simulink model "espresso_pid_wired_model_2023a"  (R2023a)
settings: Solver=VariableStepAuto  StartTime=0.0  StopTime=10  RelTol=1e-3
libraries: simulink x4, slpidlib x3
settings Model: Creator=nikonatsoulas  LastModifiedBy=Lillian K

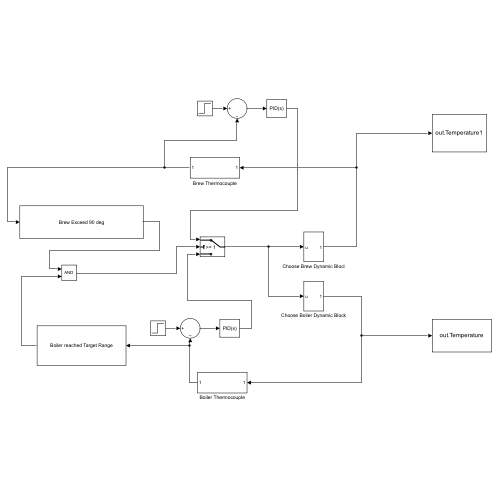
[thumbnail: Simulink's stored preview of the top-level diagram]
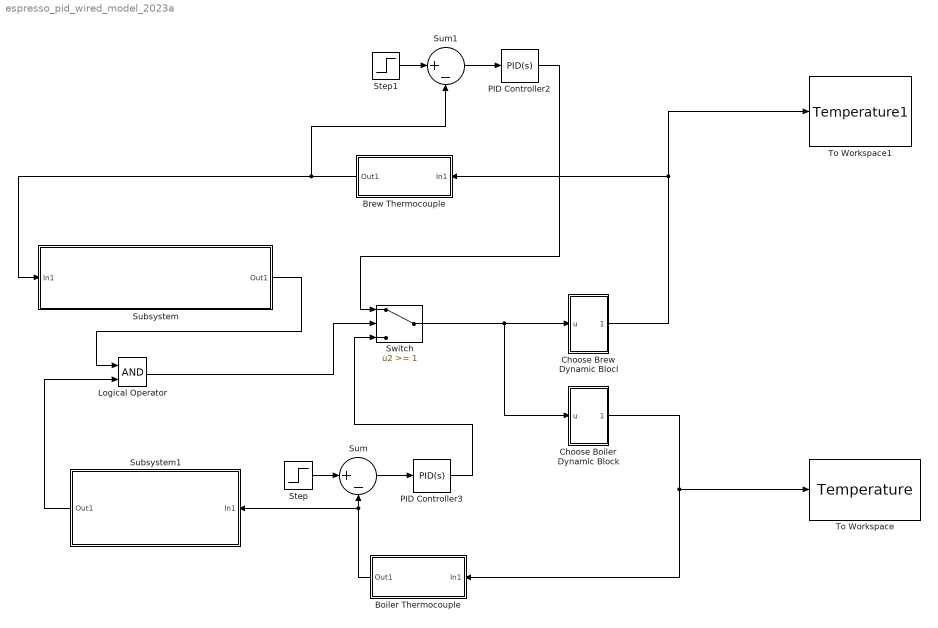
== system espresso_pid_wired_model_2023a ==
  Boiler Thermocouple : Subsystem
  Brew Thermocouple : Subsystem
  Choose Boiler Dynamic Block : Subsystem
  Choose Brew Dynamic Blocl : Subsystem
  Logical Operator : Logic  AllPortsSameDT=off  OutDataTypeStr=boolean
  PID Controller2 : slpidlib/PID Controller  Controller=PID  Form=Parallel  TimeDomain=Continuous-time  UseExternalTs=off  SampleTime=-1  IntegratorMethod=Forward Euler  FilterMethod=Forward Euler  ControllerParametersSource=internal  P=1.2  I=0.078  UseKiTs=off  D=0.08  N=100  UseFilter=on  TunerSelectOption=Transfer Function Based (PID Tuner App)  InitialConditionSource=internal  InitialConditionForIntegrator=0  InitialConditionForFilter=0  DifferentiatorICPrevScaledInput=0  ExternalReset=none  TrackingMode=off  Kt=1  LimitOutput=off  SatLimitsSource=internal  UpperSaturationLimit=inf  LowerSaturationLimit=-inf  LinearizeAsGain=on  AntiWindupMode=none  Kb=1  LimitIntegrator=off  UpperIntegratorSaturationLimit=inf  LowerIntegratorSaturationLimit=-inf  POutMin=[]  POutMax=[]  IOutMin=[]  IOutMax=[]  DOutMin=[]  DOutMax=[]  NOutMin=[]  NOutMax=[]  SumOutMin=[]  SumOutMax=[]  SaturationOutMin=[]  SaturationOutMax=[]  PParamMin=[]  PParamMax=[]  IParamMin=[]  IParamMax=[]  DParamMin=[]  DParamMax=[]  NParamMin=[]  NParamMax=[]  KbParamMin=[]  KbParamMax=[]  KtParamMin=[]  KtParamMax=[]  KbOutMin=[]  KbOutMax=[]  KtOutMin=[]  KtOutMax=[]  IntegratorOutMin=[]  IntegratorOutMax=[]  FilterOutMin=[]  FilterOutMax=[]  SumI1OutMin=[]  SumI1OutMax=[]  SumI2OutMin=[]  SumI2OutMax=[]  SumI3OutMin=[]  SumI3OutMax=[]  SumI4OutMin=[]  SumI4OutMax=[]  SumDOutMin=[]  SumDOutMax=[]  DifferentiatorOutMin=[]  DifferentiatorOutMax=[]  FilterDiffOutCoefMin=[]  FilterDiffOutCoefMax=[]  ReciprocalOutMin=[]  ReciprocalOutMax=[]  SumDenOutMin=[]  SumDenOutMax=[]  SumNumOutMin=[]  SumNumOutMax=[]  DivideOutMin=[]  DivideOutMax=[]  UdiffTsProdOutMin=[]  UdiffTsProdOutMax=[]  NTsProdOutMin=[]  NTsProdOutMax=[]  UintegralTsProdOutMin=[]  UintegralTsProdOutMax=[]  UngainTsProdOutMin=[]  UngainTsProdOutMax=[]  ClampingZeroOutDataTypeStr=Inherit: Inherit via back propagation  ClampingZeroOutMin=[]  ClampingZeroOutMax=[]  FilterDenConstantOutDataTypeStr=Inherit: Inherit via back propagation  FilterDenConstantOutMin=[]  FilterDenConstantOutMax=[]  PCopyOutDataTypeStr=Inherit: Inherit via back propagation  PCopyOutMin=[]  PCopyOutMax=[]  NCopyOutDataTypeStr=Inherit: Inherit via back propagation  NCopyOutMin=[]  NCopyOutMax=[]  IntegratorContinuousStateAttributes=''  IntegratorStateMustResolveToSignalObject=off  IntegratorRTWStateStorageClass=Auto  FilterContinuousStateAttributes=''  FilterStateMustResolveToSignalObject=off  FilterRTWStateStorageClass=Auto  ParallelPVariant=InternalParameters  IdealPVariant=Disabled  IVariant=InternalParameters  DVariant=InternalParameters  IntegratorVariant=Continuous  SatVariant=Disabled  AWVariant=Passthrough  PCopyVariant=Disabled  TRVariant=Disabled  FdbkBlocksVariant=Forward  IdealPFdbkVariant=Disabled  SatFdbkVariant=Disabled  DerivativeFilterVariant=ContFilter  NVariant=InternalParameters  NCopyVariant=Disabled  FilterICVariant=InternalICsFilter  IntegratorICVariant=InternalICs  ExternalResetVariant=Disabled  TRSumVariant=Passthrough  SumFdbkVariant=Disabled  SumVariant=Sum_PID  TsampFilterVariant=InternalTs  TsampNgainVariant=Passthrough  TsampIntegralVariant=Disabled_SignalSpec  ExternalSaturationOutDataTypeStr=Inherit: Same as second input
  PID Controller3 : slpidlib/PID Controller  Controller=PID  Form=Parallel  TimeDomain=Continuous-time  UseExternalTs=off  SampleTime=-1  IntegratorMethod=Forward Euler  FilterMethod=Forward Euler  ControllerParametersSource=internal  P=1.2  I=0.078  UseKiTs=off  D=0.08  N=100  UseFilter=on  TunerSelectOption=Transfer Function Based (PID Tuner App)  InitialConditionSource=internal  InitialConditionForIntegrator=0  InitialConditionForFilter=0  DifferentiatorICPrevScaledInput=0  ExternalReset=none  TrackingMode=off  Kt=1  LimitOutput=off  SatLimitsSource=internal  UpperSaturationLimit=inf  LowerSaturationLimit=-inf  LinearizeAsGain=on  AntiWindupMode=none  Kb=1  LimitIntegrator=off  UpperIntegratorSaturationLimit=inf  LowerIntegratorSaturationLimit=-inf  POutMin=[]  POutMax=[]  IOutMin=[]  IOutMax=[]  DOutMin=[]  DOutMax=[]  NOutMin=[]  NOutMax=[]  SumOutMin=[]  SumOutMax=[]  SaturationOutMin=[]  SaturationOutMax=[]  PParamMin=[]  PParamMax=[]  IParamMin=[]  IParamMax=[]  DParamMin=[]  DParamMax=[]  NParamMin=[]  NParamMax=[]  KbParamMin=[]  KbParamMax=[]  KtParamMin=[]  KtParamMax=[]  KbOutMin=[]  KbOutMax=[]  KtOutMin=[]  KtOutMax=[]  IntegratorOutMin=[]  IntegratorOutMax=[]  FilterOutMin=[]  FilterOutMax=[]  SumI1OutMin=[]  SumI1OutMax=[]  SumI2OutMin=[]  SumI2OutMax=[]  SumI3OutMin=[]  SumI3OutMax=[]  SumI4OutMin=[]  SumI4OutMax=[]  SumDOutMin=[]  SumDOutMax=[]  DifferentiatorOutMin=[]  DifferentiatorOutMax=[]  FilterDiffOutCoefMin=[]  FilterDiffOutCoefMax=[]  ReciprocalOutMin=[]  ReciprocalOutMax=[]  SumDenOutMin=[]  SumDenOutMax=[]  SumNumOutMin=[]  SumNumOutMax=[]  DivideOutMin=[]  DivideOutMax=[]  UdiffTsProdOutMin=[]  UdiffTsProdOutMax=[]  NTsProdOutMin=[]  NTsProdOutMax=[]  UintegralTsProdOutMin=[]  UintegralTsProdOutMax=[]  UngainTsProdOutMin=[]  UngainTsProdOutMax=[]  ClampingZeroOutDataTypeStr=Inherit: Inherit via back propagation  ClampingZeroOutMin=[]  ClampingZeroOutMax=[]  FilterDenConstantOutDataTypeStr=Inherit: Inherit via back propagation  FilterDenConstantOutMin=[]  FilterDenConstantOutMax=[]  PCopyOutDataTypeStr=Inherit: Inherit via back propagation  PCopyOutMin=[]  PCopyOutMax=[]  NCopyOutDataTypeStr=Inherit: Inherit via back propagation  NCopyOutMin=[]  NCopyOutMax=[]  IntegratorContinuousStateAttributes=''  IntegratorStateMustResolveToSignalObject=off  IntegratorRTWStateStorageClass=Auto  FilterContinuousStateAttributes=''  FilterStateMustResolveToSignalObject=off  FilterRTWStateStorageClass=Auto  ParallelPVariant=InternalParameters  IdealPVariant=Disabled  IVariant=InternalParameters  DVariant=InternalParameters  IntegratorVariant=Continuous  SatVariant=Disabled  AWVariant=Passthrough  PCopyVariant=Disabled  TRVariant=Disabled  FdbkBlocksVariant=Forward  IdealPFdbkVariant=Disabled  SatFdbkVariant=Disabled  DerivativeFilterVariant=ContFilter  NVariant=InternalParameters  NCopyVariant=Disabled  FilterICVariant=InternalICsFilter  IntegratorICVariant=InternalICs  ExternalResetVariant=Disabled  TRSumVariant=Passthrough  SumFdbkVariant=Disabled  SumVariant=Sum_PID  TsampFilterVariant=InternalTs  TsampNgainVariant=Passthrough  TsampIntegralVariant=Disabled_SignalSpec  ExternalSaturationOutDataTypeStr=Inherit: Same as second input
  Step : Step  After=65  SampleTime=0
  Step1 : Step  SampleTime=0
  Subsystem : Subsystem
      mask Display: disp('Brew Exceed 90 deg')
  Subsystem1 : Subsystem
      mask Display: disp('Boiler reached Target Range')
  Sum : Sum  Inputs=|+-
  Sum1 : Sum  Inputs=|+-
  Switch : Switch  Threshold=1  SaturateOnIntegerOverflow=off  InputSameDT=off
  To Workspace : ToWorkspace  VariableName=Temperature  SaveFormat=Timeseries  SampleTime=-1
  To Workspace1 : ToWorkspace  VariableName=Temperature1  SaveFormat=Timeseries  SampleTime=-1
  wires:
  Step/1 -> Sum/1
  Boiler Thermocouple/1(Out1) -> Sum/2, Subsystem1/1(In1)
  Step1/1 -> Sum1/1
  Brew Thermocouple/1(Out1) -> Sum1/2, Subsystem/1(In1)
  PID Controller2/1 -> Switch/1
  PID Controller3/1 -> Switch/3
  Logical Operator/1 -> Switch/2
  Sum/1 -> PID Controller3/1
  Switch/1 -> Choose Brew Dynamic Blocl/1(u), Choose Boiler Dynamic Block/1(u)
  Sum1/1 -> PID Controller2/1
  Choose Boiler Dynamic Block/1(Out1) -> Boiler Thermocouple/1(In1), To Workspace/1
  Choose Brew Dynamic Blocl/1(Out1) -> To Workspace1/1, Brew Thermocouple/1(In1)
  Subsystem/1(Out1) -> Logical Operator/1
  Subsystem1/1(Out1) -> Logical Operator/2

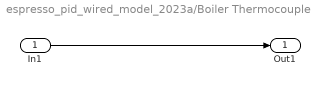
== system espresso_pid_wired_model_2023a/Boiler Thermocouple ==
  In1 : Inport
  Out1 : Outport
  wires:
  In1/1 -> Out1/1

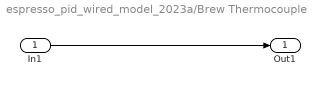
== system espresso_pid_wired_model_2023a/Brew Thermocouple ==
  In1 : Inport
  Out1 : Outport
  wires:
  In1/1 -> Out1/1

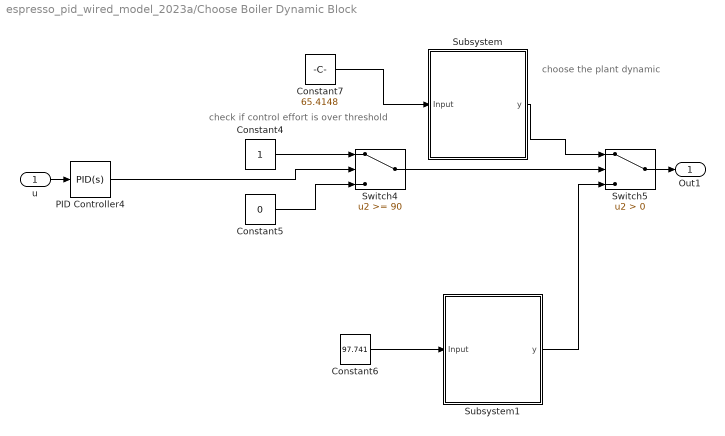
== system espresso_pid_wired_model_2023a/Choose Boiler Dynamic Block ==
  note: choose the plant dynamic
  note: check if control effort is over threshold
  u : Inport
  Constant4 : Constant
  Constant5 : Constant  Value=0
  Constant6 : Constant  Value=97.741
  Constant7 : Constant  Value=65.4148
  PID Controller4 : slpidlib/PID Controller  Controller=PID  Form=Parallel  TimeDomain=Continuous-time  UseExternalTs=off  SampleTime=-1  IntegratorMethod=Forward Euler  FilterMethod=Forward Euler  ControllerParametersSource=internal  P=1.2  I=0.078  UseKiTs=off  D=0.08  N=100  UseFilter=on  TunerSelectOption=Transfer Function Based (PID Tuner App)  InitialConditionSource=internal  InitialConditionForIntegrator=0  InitialConditionForFilter=0  DifferentiatorICPrevScaledInput=0  ExternalReset=none  TrackingMode=off  Kt=1  LimitOutput=off  SatLimitsSource=internal  UpperSaturationLimit=inf  LowerSaturationLimit=-inf  LinearizeAsGain=on  AntiWindupMode=none  Kb=1  LimitIntegrator=off  UpperIntegratorSaturationLimit=inf  LowerIntegratorSaturationLimit=-inf  POutMin=[]  POutMax=[]  IOutMin=[]  IOutMax=[]  DOutMin=[]  DOutMax=[]  NOutMin=[]  NOutMax=[]  SumOutMin=[]  SumOutMax=[]  SaturationOutMin=[]  SaturationOutMax=[]  PParamMin=[]  PParamMax=[]  IParamMin=[]  IParamMax=[]  DParamMin=[]  DParamMax=[]  NParamMin=[]  NParamMax=[]  KbParamMin=[]  KbParamMax=[]  KtParamMin=[]  KtParamMax=[]  KbOutMin=[]  KbOutMax=[]  KtOutMin=[]  KtOutMax=[]  IntegratorOutMin=[]  IntegratorOutMax=[]  FilterOutMin=[]  FilterOutMax=[]  SumI1OutMin=[]  SumI1OutMax=[]  SumI2OutMin=[]  SumI2OutMax=[]  SumI3OutMin=[]  SumI3OutMax=[]  SumI4OutMin=[]  SumI4OutMax=[]  SumDOutMin=[]  SumDOutMax=[]  DifferentiatorOutMin=[]  DifferentiatorOutMax=[]  FilterDiffOutCoefMin=[]  FilterDiffOutCoefMax=[]  ReciprocalOutMin=[]  ReciprocalOutMax=[]  SumDenOutMin=[]  SumDenOutMax=[]  SumNumOutMin=[]  SumNumOutMax=[]  DivideOutMin=[]  DivideOutMax=[]  UdiffTsProdOutMin=[]  UdiffTsProdOutMax=[]  NTsProdOutMin=[]  NTsProdOutMax=[]  UintegralTsProdOutMin=[]  UintegralTsProdOutMax=[]  UngainTsProdOutMin=[]  UngainTsProdOutMax=[]  ClampingZeroOutDataTypeStr=Inherit: Inherit via back propagation  ClampingZeroOutMin=[]  ClampingZeroOutMax=[]  FilterDenConstantOutDataTypeStr=Inherit: Inherit via back propagation  FilterDenConstantOutMin=[]  FilterDenConstantOutMax=[]  PCopyOutDataTypeStr=Inherit: Inherit via back propagation  PCopyOutMin=[]  PCopyOutMax=[]  NCopyOutDataTypeStr=Inherit: Inherit via back propagation  NCopyOutMin=[]  NCopyOutMax=[]  IntegratorContinuousStateAttributes=''  IntegratorStateMustResolveToSignalObject=off  IntegratorRTWStateStorageClass=Auto  FilterContinuousStateAttributes=''  FilterStateMustResolveToSignalObject=off  FilterRTWStateStorageClass=Auto  ParallelPVariant=InternalParameters  IdealPVariant=Disabled  IVariant=InternalParameters  DVariant=InternalParameters  IntegratorVariant=Continuous  SatVariant=Disabled  AWVariant=Passthrough  PCopyVariant=Disabled  TRVariant=Disabled  FdbkBlocksVariant=Forward  IdealPFdbkVariant=Disabled  SatFdbkVariant=Disabled  DerivativeFilterVariant=ContFilter  NVariant=InternalParameters  NCopyVariant=Disabled  FilterICVariant=InternalICsFilter  IntegratorICVariant=InternalICs  ExternalResetVariant=Disabled  TRSumVariant=Passthrough  SumFdbkVariant=Disabled  SumVariant=Sum_PID  TsampFilterVariant=InternalTs  TsampNgainVariant=Passthrough  TsampIntegralVariant=Disabled_SignalSpec  ExternalSaturationOutDataTypeStr=Inherit: Same as second input
  Subsystem : Subsystem
      mask Display: disp('Full 40 A to Brew')
  Subsystem1 : Subsystem
      mask Display: disp('0 A to Brew')
  Switch4 : Switch  Threshold=90  SaturateOnIntegerOverflow=off  InputSameDT=off
  Switch5 : Switch  Criteria=u2 > Threshold  SaturateOnIntegerOverflow=off  InputSameDT=off
  Out1 : Outport
  wires:
  Constant5/1 -> Switch4/3
  Switch4/1 -> Switch5/2
  PID Controller4/1 -> Switch4/2
  Constant6/1 -> Subsystem1/1(Input)
  Constant7/1 -> Subsystem/1(Input)
  Constant4/1 -> Switch4/1
  Subsystem/1(y) -> Switch5/1
  Subsystem1/1(y) -> Switch5/3
  Switch5/1 -> Out1/1
  u/1 -> PID Controller4/1

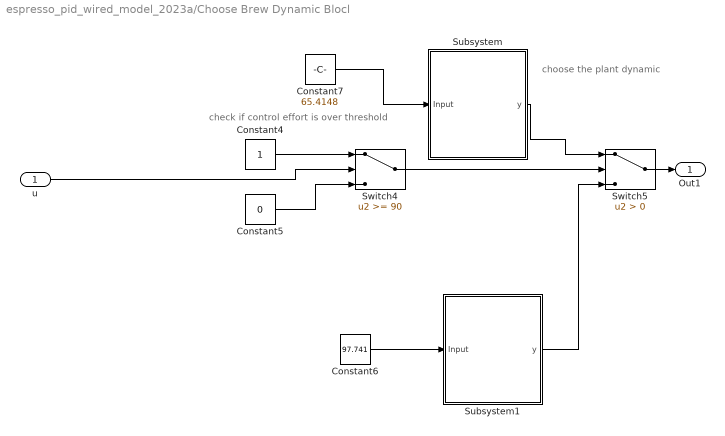
== system espresso_pid_wired_model_2023a/Choose Brew Dynamic Blocl ==
  note: choose the plant dynamic
  note: check if control effort is over threshold
  u : Inport
  Constant4 : Constant
  Constant5 : Constant  Value=0
  Constant6 : Constant  Value=97.741
  Constant7 : Constant  Value=65.4148
  Subsystem : Subsystem
      mask Display: disp('Full 40 A to Brew')
  Subsystem1 : Subsystem
      mask Display: disp('0 A to Brew')
  Switch4 : Switch  Threshold=90  SaturateOnIntegerOverflow=off  InputSameDT=off
  Switch5 : Switch  Criteria=u2 > Threshold  SaturateOnIntegerOverflow=off  InputSameDT=off
  Out1 : Outport
  wires:
  Constant5/1 -> Switch4/3
  Switch4/1 -> Switch5/2
  u/1 -> Switch4/2
  Constant6/1 -> Subsystem1/1(Input)
  Constant7/1 -> Subsystem/1(Input)
  Constant4/1 -> Switch4/1
  Subsystem/1(y) -> Switch5/1
  Subsystem1/1(y) -> Switch5/3
  Switch5/1 -> Out1/1

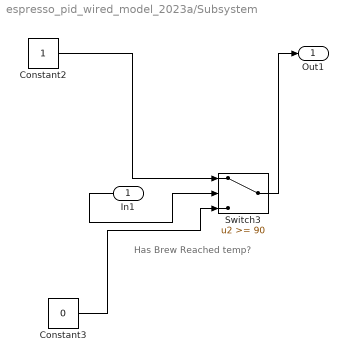
== system espresso_pid_wired_model_2023a/Subsystem ==
  note: Has Brew Reached temp?
  In1 : Inport
  Constant2 : Constant
  Constant3 : Constant  Value=0
  Switch3 : Switch  Threshold=90  SaturateOnIntegerOverflow=off  InputSameDT=off
  Out1 : Outport
  wires:
  Constant2/1 -> Switch3/1
  Switch3/1 -> Out1/1
  Constant3/1 -> Switch3/3
  In1/1 -> Switch3/2

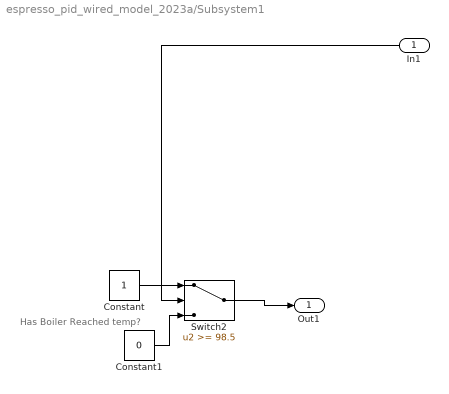
== system espresso_pid_wired_model_2023a/Subsystem1 ==
  note: Has Boiler Reached temp?
  In1 : Inport
  Constant : Constant
  Constant1 : Constant  Value=0
  Switch2 : Switch  Threshold=98.5  SaturateOnIntegerOverflow=off  InputSameDT=off
  Out1 : Outport
  wires:
  Constant/1 -> Switch2/1
  Constant1/1 -> Switch2/3
  In1/1 -> Switch2/2
  Switch2/1 -> Out1/1

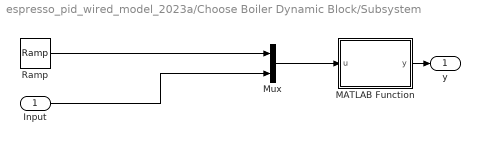
== system espresso_pid_wired_model_2023a/Choose Boiler Dynamic Block/Subsystem ==
  Input : Inport
  MATLAB Function : MATLAB Function  TreatAsAtomicUnit=on
  Mux : Mux  Inputs=2
  Ramp : simulink/Sources/Ramp  slope=1  start=0  InitialOutput=0
  y : Outport
  wires:
  Ramp/1 -> Mux/1
  MATLAB Function/1(y) -> y/1
  Mux/1 -> MATLAB Function/1(u)
  Input/1 -> Mux/2

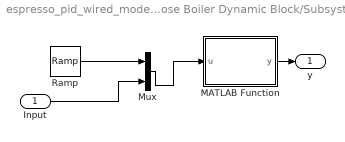
== system espresso_pid_wired_model_2023a/Choose Boiler Dynamic Block/Subsystem1 ==
  Input : Inport
  MATLAB Function : MATLAB Function  TreatAsAtomicUnit=on
  Mux : Mux  Inputs=2
  Ramp : simulink/Sources/Ramp  slope=1  start=0  InitialOutput=0
  y : Outport
  wires:
  MATLAB Function/1(y) -> y/1
  Input/1 -> Mux/2
  Mux/1 -> MATLAB Function/1(u)
  Ramp/1 -> Mux/1

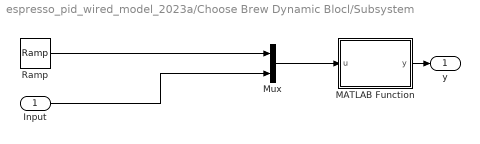
== system espresso_pid_wired_model_2023a/Choose Brew Dynamic Blocl/Subsystem ==
  Input : Inport
  MATLAB Function : MATLAB Function  TreatAsAtomicUnit=on
  Mux : Mux  Inputs=2
  Ramp : simulink/Sources/Ramp  slope=1  start=0  InitialOutput=0
  y : Outport
  wires:
  Ramp/1 -> Mux/1
  MATLAB Function/1(y) -> y/1
  Mux/1 -> MATLAB Function/1(u)
  Input/1 -> Mux/2

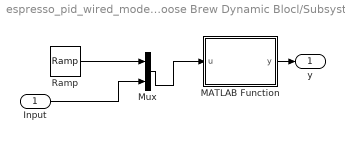
== system espresso_pid_wired_model_2023a/Choose Brew Dynamic Blocl/Subsystem1 ==
  Input : Inport
  MATLAB Function : MATLAB Function  TreatAsAtomicUnit=on
  Mux : Mux  Inputs=2
  Ramp : simulink/Sources/Ramp  slope=1  start=0  InitialOutput=0
  y : Outport
  wires:
  MATLAB Function/1(y) -> y/1
  Input/1 -> Mux/2
  Mux/1 -> MATLAB Function/1(u)
  Ramp/1 -> Mux/1

== matlab function espresso_pid_wired_model_2023a/Choose Brew Dynamic Blocl/Subsystem/MATLAB Function ==
  data: u input; y output
function y = fcn(u)

y = 0.0006 * u(1)^2 + 0.1766 * u(1) +u(2);
end

== matlab function espresso_pid_wired_model_2023a/Choose Boiler Dynamic Block/Subsystem/MATLAB Function ==
  data: u input; y output
function y = fcn(u)

y = 0.0006 * u(1)^2 + 0.1766 * u(1) +u(2);
end

== matlab function espresso_pid_wired_model_2023a/Choose Boiler Dynamic Block/Subsystem1/MATLAB Function ==
  data: u input; y output
function y = fcn(u)

y = 0.0172 * u(1)^2 + -0.6276 * u(1) + u(2);
end

== matlab function espresso_pid_wired_model_2023a/Choose Brew Dynamic Blocl/Subsystem1/MATLAB Function ==
  data: u input; y output
function y = fcn(u)

y = 0.0172 * u(1)^2 + -0.6276 * u(1) + u(2);
end
